simulink library "addedMassFuseOnly_cl"  (R2022a)
settings: Solver=VariableStepAuto  StartTime=0.0  StopTime=10.0  RelTol=1e-3
undefined symbols (not defined in the file): vcl
libraries: xProdMatrix_ul x3, vrlib x1
settings Model: Creator=jldanie5  LastModifiedBy=adabney
settings SolverCC: AlgebraicLoopSolver=TrustRegion
settings DebuggingCC: UnconnectedInputMsg=warning  UnconnectedOutputMsg=warning  UnconnectedLineMsg=warning  SFMachineParentedDataDiag=warning  ArithmeticOperatorsInVariantConditions=warning
settings SFSimCC: CustomCodeUndefinedFunction=UseInterfaceOnly

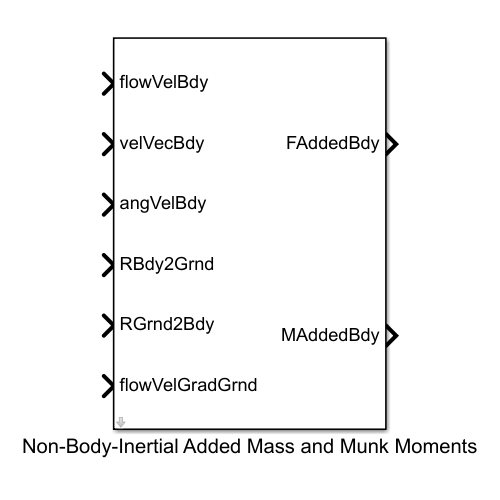
[thumbnail: Simulink's stored preview of the top-level diagram]
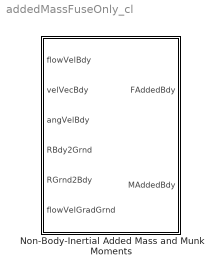
== system addedMassFuseOnly_cl ==
  Non-Body-Inertial Added Mass and Munk Moments : Subsystem  mask{MaMat=vcl.Ma6x6_LE.Value, MaMatFuse=vcl.Ma6x6_LE_Fuse.Value, rB_LE=vcl.rB_LE.Value, gradDist=vcl.flowGradientDist.Value}
      mask prompts: MaMat "Kite Added Mass Matrix"; MaMatFuse "Fuselage Added Mass Matrix"; rB_LE "Body frame origin position relative to the leading edge"; gradDist "Gradient Spacial Distance"
      mask init:
      | S=@(v) [0 -v(3) v(2);v(3) 0 -v(1);-v(2) v(1) 0];
      | MaAdj = [eye(3) zeros(3);-S(rB_LE) eye(3)];

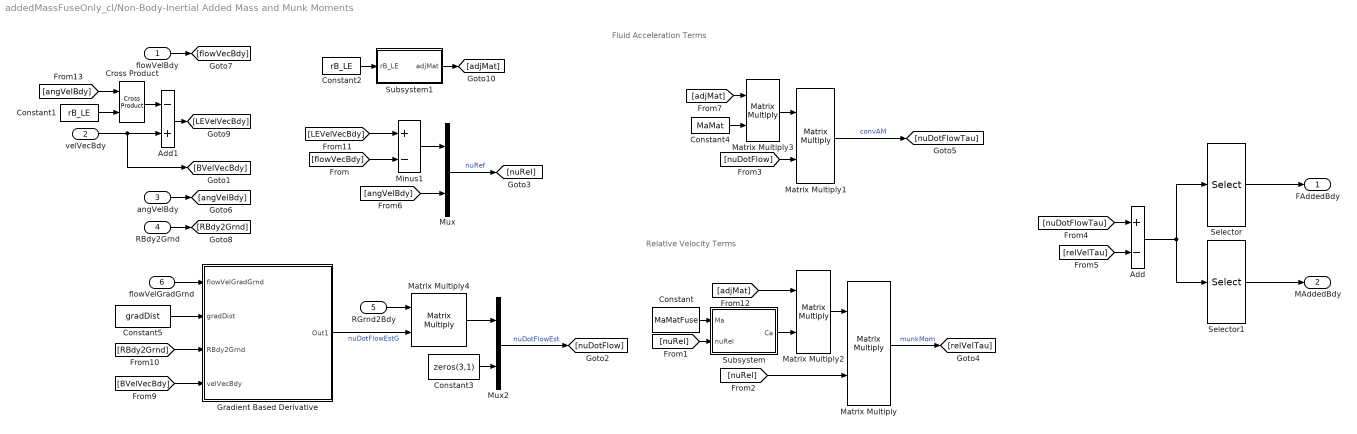
== system addedMassFuseOnly_cl/Non-Body-Inertial Added Mass and Munk Moments ==
  note: Fluid Acceleration Terms
  note: Relative Velocity Terms
  "flowVelBdy " : Inport
  velVecBdy : Inport  Port=2
  angVelBdy : Inport  Port=3
  RBdy2Grnd : Inport  Port=4
  RGrnd2Bdy : Inport  Port=5
  flowVelGradGrnd : Inport  Port=6
  Add : Sum  Inputs=+-
  Add1 : Sum  Inputs=-+
  Constant : Constant  Value=MaMatFuse
  Constant1 : Constant  Value=rB_LE
  Constant2 : Constant  Value=rB_LE
  Constant3 : Constant  Value=zeros(3,1)
  Constant4 : Constant  Value=MaMat
  Constant5 : Constant  Value=gradDist
  Cross Product : vrlib/Utilities/Cross Product
  Gradient Based Derivative : Subsystem
  Matrix Multiply{,1..4} (5 alike) : Product  Multiplication=Matrix(*)
  Minus1 : Sum  Inputs=+-
  Mux : Mux  Inputs=2
  Mux2 : Mux  Inputs=2
  Selector : Selector  InputPortWidth=6  IndexOptions=Index vector (dialog)  Indices=[1 2 3]  OutputSizes=1
  Selector1 : Selector  InputPortWidth=6  IndexOptions=Index vector (dialog)  Indices=[4 5 6]  OutputSizes=1
  Subsystem : Subsystem
  Subsystem1 : Subsystem
  FAddedBdy : Outport  VectorParamsAs1DForOutWhenUnconnected=off
  MAddedBdy : Outport  Port=2  VectorParamsAs1DForOutWhenUnconnected=off
  wires:
  Gradient Based Derivative/1(Out1) -> Matrix Multiply4/2  "nuDotFlowEstG"
  RBdy2Grnd/1 -> [RBdy2Grnd]
  [BVelVecBdy] -> Gradient Based Derivative/4(velVecBdy)
  [RBdy2Grnd] -> Gradient Based Derivative/3(RBdy2Grnd)
  Constant5/1 -> Gradient Based Derivative/2(gradDist)
  flowVelGradGrnd/1 -> Gradient Based Derivative/1(flowVelGradGrnd)
  velVecBdy/1 -> Add1/2, [BVelVecBdy]
  Mux/1 -> [nuRel]  "nuRef"
  Minus1/1 -> Mux/1
  Matrix Multiply4/1 -> Mux2/1
  RGrnd2Bdy/1 -> Matrix Multiply4/1
  Mux2/1 -> [nuDotFlow]  "nuDotFlowEst"
  Constant3/1 -> Mux2/2
  Add/1 -> Selector1/1, Selector/1
  [nuDotFlowTau] -> Add/1
  [relVelTau] -> Add/2
  Matrix Multiply1/1 -> [nuDotFlowTau]  "convAM"
  [nuDotFlow] -> Matrix Multiply1/2
  Matrix Multiply3/1 -> Matrix Multiply1/1
  Matrix Multiply/1 -> [relVelTau]  "munkMom"
  [nuRel] -> Matrix Multiply/2
  [nuRel] -> Subsystem/2(nuRel)
  Constant/1 -> Subsystem/1(Ma)
  "flowVelBdy "/1 -> [flowVecBdy]
  angVelBdy/1 -> [angVelBdy]
  [angVelBdy] -> Mux/2
  Cross Product/1 -> Add1/1
  [angVelBdy] -> Cross Product/1
  Constant1/1 -> Cross Product/2
  Add1/1 -> [LEVelVecBdy]
  [LEVelVecBdy] -> Minus1/1
  [flowVecBdy] -> Minus1/2
  [adjMat] -> Matrix Multiply2/1
  Subsystem/1(Ca) -> Matrix Multiply2/2
  Matrix Multiply2/1 -> Matrix Multiply/1
  [adjMat] -> Matrix Multiply3/1
  Constant4/1 -> Matrix Multiply3/2
  Constant2/1 -> Subsystem1/1(rB_LE)
  Subsystem1/1(adjMat) -> [adjMat]
  Selector/1 -> FAddedBdy/1
  Selector1/1 -> MAddedBdy/1

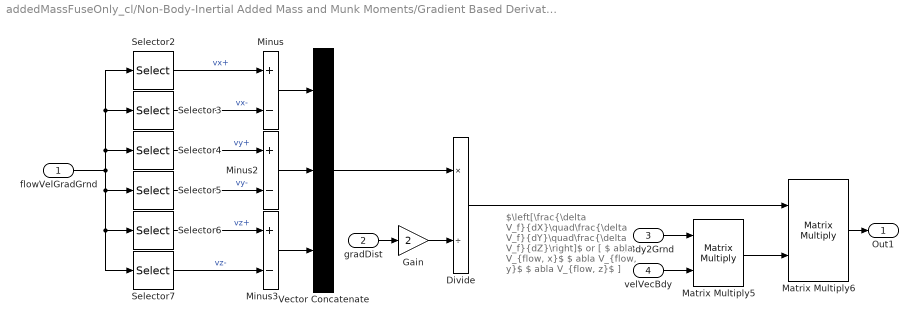
== system addedMassFuseOnly_cl/Non-Body-Inertial Added Mass and Munk Moments/Gradient Based Derivative ==
  note: $\left[\frac{\delta V_f}{dX}\quad\frac{\delta V_f}{dY}\quad\frac{\delta V_f}{dZ}\right]$
      | or
      | [ $\nabla V_{flow, x}$
      | $\nabla V_{flow, y}$
      | $\nabla V_{flow, z}$ ]
  flowVelGradGrnd : Inport
  gradDist : Inport  Port=2
  RBdy2Grnd : Inport  Port=3
  velVecBdy : Inport  Port=4
  Divide : Product  Inputs=*/
  Gain : Gain  Gain=2
  Matrix Multiply5 : Product  Multiplication=Matrix(*)
  Matrix Multiply6 : Product  Multiplication=Matrix(*)
  Minus : Sum  Inputs=+-
  Minus2 : Sum  Inputs=+-
  Minus3 : Sum  Inputs=+-
  Selector2 : Selector  NumberOfDimensions=2  InputPortWidth=3  IndexOptions=Select all,Index vector (dialog)  Indices=[1 3],1  OutputSizes=1,1
  Selector3 : Selector  NumberOfDimensions=2  InputPortWidth=3  IndexOptions=Select all,Index vector (dialog)  Indices=[1 3],4  OutputSizes=1,1
  Selector4 : Selector  NumberOfDimensions=2  InputPortWidth=3  IndexOptions=Select all,Index vector (dialog)  Indices=[1 3],2  OutputSizes=1,1
  Selector5 : Selector  NumberOfDimensions=2  InputPortWidth=3  IndexOptions=Select all,Index vector (dialog)  Indices=[1 3],5  OutputSizes=1,1
  Selector6 : Selector  NumberOfDimensions=2  InputPortWidth=3  IndexOptions=Select all,Index vector (dialog)  Indices=[1 3],3  OutputSizes=1,1
  Selector7 : Selector  NumberOfDimensions=2  InputPortWidth=3  IndexOptions=Select all,Index vector (dialog)  Indices=[1 3],1  OutputSizes=1,1
  Vector Concatenate : Concatenate  NumInputs=3  Mode=Multidimensional array  ConcatenateDimension=2
  Out1 : Outport  VectorParamsAs1DForOutWhenUnconnected=off
  wires:
  Matrix Multiply6/1 -> Out1/1
  Divide/1 -> Matrix Multiply6/1
  Selector2/1 -> Minus/1  "vx+"
  Selector3/1 -> Minus/2  "vx-"
  RBdy2Grnd/1 -> Matrix Multiply5/1
  Gain/1 -> Divide/2
  Minus3/1 -> Vector Concatenate/3
  flowVelGradGrnd/1 -> Selector7/1, Selector6/1, Selector5/1, Selector2/1, Selector3/1, Selector4/1
  Selector5/1 -> Minus2/2  "vy-"
  gradDist/1 -> Gain/1
  Selector4/1 -> Minus2/1  "vy+"
  Selector6/1 -> Minus3/1  "vz+"
  Vector Concatenate/1 -> Divide/1
  Minus2/1 -> Vector Concatenate/2
  Selector7/1 -> Minus3/2  "vz-"
  Matrix Multiply5/1 -> Matrix Multiply6/2
  Minus/1 -> Vector Concatenate/1
  velVecBdy/1 -> Matrix Multiply5/2

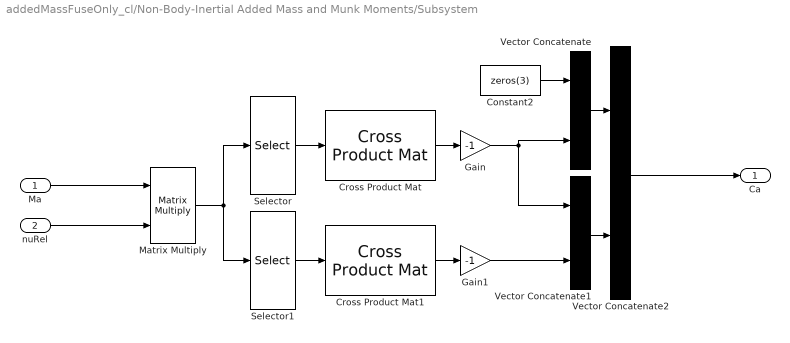
== system addedMassFuseOnly_cl/Non-Body-Inertial Added Mass and Munk Moments/Subsystem ==
  Ma : Inport
  nuRel : Inport  Port=2
  Constant2 : Constant  Value=zeros(3)
  Cross Product Mat : xProdMatrix_ul/Cross Product Mat  SystemSampleTime=-1  VariantActivationTime=update diagram  Latency=0  AutoFrameSizeCalculation=off
  Cross Product Mat1 : xProdMatrix_ul/Cross Product Mat  SystemSampleTime=-1  VariantActivationTime=update diagram  Latency=0  AutoFrameSizeCalculation=off
  Gain : Gain  Gain=-1
  Gain1 : Gain  Gain=-1
  Matrix Multiply : Product  Multiplication=Matrix(*)
  Selector : Selector  InputPortWidth=6  IndexOptions=Index vector (dialog)  Indices=[1 2 3]  OutputSizes=1
  Selector1 : Selector  InputPortWidth=6  IndexOptions=Index vector (dialog)  Indices=[4 5 6]  OutputSizes=1
  Vector Concatenate : Concatenate  Mode=Multidimensional array  ConcatenateDimension=2
  Vector Concatenate1 : Concatenate  Mode=Multidimensional array  ConcatenateDimension=2
  Vector Concatenate2 : Concatenate  Mode=Multidimensional array
  Ca : Outport  VectorParamsAs1DForOutWhenUnconnected=off
  wires:
  Vector Concatenate2/1 -> Ca/1
  nuRel/1 -> Matrix Multiply/2
  Constant2/1 -> Vector Concatenate/1
  Vector Concatenate/1 -> Vector Concatenate2/1
  Gain1/1 -> Vector Concatenate1/2
  Cross Product Mat/1 -> Gain/1
  Vector Concatenate1/1 -> Vector Concatenate2/2
  Cross Product Mat1/1 -> Gain1/1
  Selector1/1 -> Cross Product Mat1/1
  Matrix Multiply/1 -> Selector1/1, Selector/1
  Selector/1 -> Cross Product Mat/1
  Ma/1 -> Matrix Multiply/1
  Gain/1 -> Vector Concatenate/2, Vector Concatenate1/1

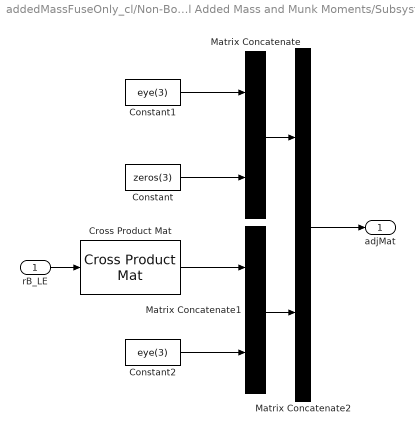
== system addedMassFuseOnly_cl/Non-Body-Inertial Added Mass and Munk Moments/Subsystem1 ==
  rB_LE : Inport
  Constant : Constant  Value=zeros(3)
  Constant1 : Constant  Value=eye(3)
  Constant2 : Constant  Value=eye(3)
  Cross Product Mat : xProdMatrix_ul/Cross Product Mat  SystemSampleTime=-1  VariantActivationTime=update diagram  Latency=0  AutoFrameSizeCalculation=off
  Matrix Concatenate : Concatenate  Mode=Multidimensional array  ConcatenateDimension=2
  Matrix Concatenate1 : Concatenate  Mode=Multidimensional array  ConcatenateDimension=2
  Matrix Concatenate2 : Concatenate  Mode=Multidimensional array
  adjMat : Outport  VectorParamsAs1DForOutWhenUnconnected=off
  wires:
  Matrix Concatenate/1 -> Matrix Concatenate2/1
  Matrix Concatenate1/1 -> Matrix Concatenate2/2
  rB_LE/1 -> Cross Product Mat/1
  Cross Product Mat/1 -> Matrix Concatenate1/1
  Constant/1 -> Matrix Concatenate/2
  Constant1/1 -> Matrix Concatenate/1
  Constant2/1 -> Matrix Concatenate1/2
  Matrix Concatenate2/1 -> adjMat/1
